simulink model "PO2"  (R2023a)
settings: Solver=VariableStepAuto  StartTime=0.0  StopTime=10.0  RelTol=1e-3
settings Model: Creator=meghn  LastModifiedBy=meghn

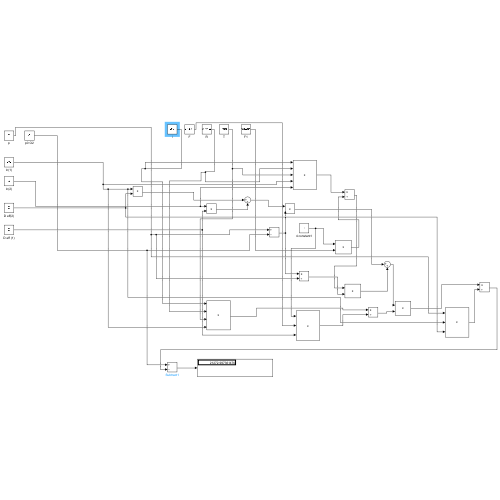
[thumbnail: Simulink's stored preview of the top-level diagram]
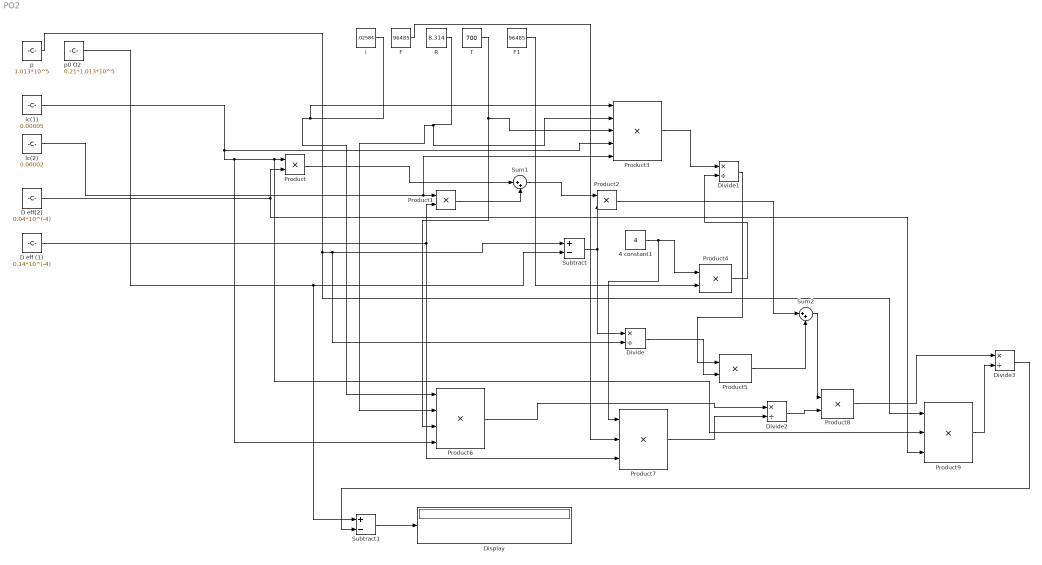
== system PO2 ==
  4 constant1 : Constant  Value=4
  D eff (1) : Constant  Value=0.14*10^(-4)
  D eff(2) : Constant  Value=0.04*10^(-4)
  Display : Display
  Divide{,1..3} (4 alike) : Product  Inputs=*/
  F : Constant  Value=96485
  F1 : Constant  Value=96485
  Product{,1..2,4..5,8} (6 alike) : Product
  Product3 : Product  Inputs=5
  Product6 : Product  Inputs=4
  Product7 : Product  Inputs=3
  Product9 : Product  Inputs=3
  R : Constant  Value=8.314
  Subtract : Sum  Inputs=+-
  Subtract1 : Sum  Inputs=+-
  Sum1 : Sum  Inputs=|++
  Sum2 : Sum  Inputs=|++
  T : Constant  Value=700
  i : Constant  Value=.02584
  lc(1) : Constant  Value=0.00005
  lc(2) : Constant  Value=0.00002
  p : Constant  Value=1.013*10^5
  p0 O2 : Constant  Value=0.21*1.013*10^5
  wires:
  D eff(2)/1 -> Product/2, Product9/3
  lc(1)/1 -> Product6/4, Product9/2, Product/1, Product3/4
  p/1 -> Product9/1, Divide/2, Subtract/1
  p0 O2/1 -> Subtract1/1, Subtract/2
  lc(2)/1 -> Product3/5, Product1/1
  D eff (1)/1 -> Product1/2, Product7/3
  Product/1 -> Sum1/1
  Product1/1 -> Sum1/2
  Sum1/1 -> Product2/1
  Subtract/1 -> Product2/2, Divide/1
  i/1 -> Product6/1, Product3/1
  R/1 -> Product6/2, Product3/2
  T/1 -> Product6/3, Product3/3
  4 constant1/1 -> Product7/1, Product4/1
  F1/1 -> Product4/2
  Product3/1 -> Divide1/1
  Product4/1 -> Divide1/2
  Divide/1 -> Product5/2
  Divide1/1 -> Product5/1
  Product2/1 -> Sum2/1
  Product5/1 -> Sum2/2
  F/1 -> Product7/2
  Product6/1 -> Divide2/1
  Product7/1 -> Divide2/2
  Sum2/1 -> Product8/1
  Divide2/1 -> Product8/2
  Product8/1 -> Divide3/1
  Product9/1 -> Divide3/2
  Divide3/1 -> Subtract1/2
  Subtract1/1 -> Display/1
